simulink model "Hibrido2"  (R2015a)
settings: Solver=ode45  StartTime=0.0  StopTime=1  RelTol=1e-3
values from neighbouring files (symbols this model uses):
  T = 1    [Variaveis.mat]
settings Model: Creator=Afonso  LastModifiedBy=Élio

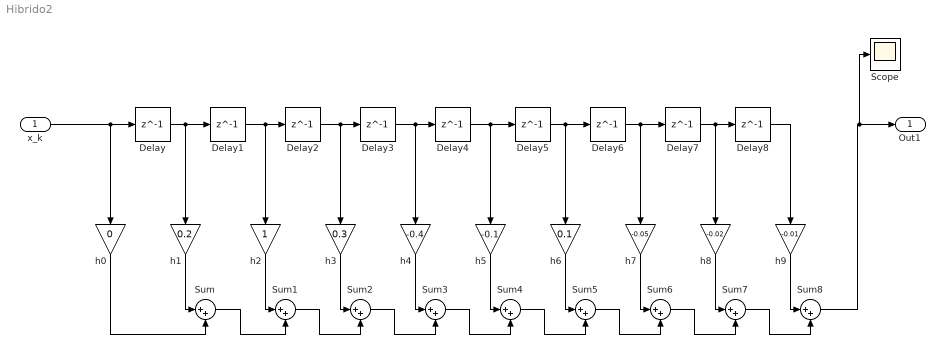
== system Hibrido2 ==
  x_k : Inport
  Delay{,1..8} (9 alike) : Delay  DelayLength=1  SampleTime=T
  Scope : Scope
  Sum{,1..8} (9 alike) : Sum  Inputs=|++
  h0 : Gain  Gain=0
  h1 : Gain  Gain=0.2
  h2 : Gain
  h3 : Gain  Gain=0.3
  h4 : Gain  Gain=-0.4
  h5 : Gain  Gain=-0.1
  h6 : Gain  Gain=0.1
  h7 : Gain  Gain=-0.05
  h8 : Gain  Gain=-0.02
  h9 : Gain  Gain=-0.01
  Out1 : Outport
  wires:
  Sum5/1 -> Sum6/2
  Sum1/1 -> Sum2/2
  Sum6/1 -> Sum7/2
  h9/1 -> Sum8/1
  Sum4/1 -> Sum5/2
  Sum7/1 -> Sum8/2
  Sum3/1 -> Sum4/2
  Sum8/1 -> Scope/1, Out1/1
  Sum2/1 -> Sum3/2
  h7/1 -> Sum6/1
  h8/1 -> Sum7/1
  Delay1/1 -> Delay2/1, h2/1
  Delay/1 -> Delay1/1, h1/1
  Delay2/1 -> Delay3/1, h3/1
  Delay3/1 -> Delay4/1, h4/1
  Delay4/1 -> Delay5/1, h5/1
  Delay6/1 -> Delay7/1, h7/1
  Sum/1 -> Sum1/2
  h2/1 -> Sum1/1
  Delay8/1 -> h9/1
  h1/1 -> Sum/1
  Delay7/1 -> Delay8/1, h8/1
  x_k/1 -> Delay/1, h0/1
  h0/1 -> Sum/2
  h4/1 -> Sum3/1
  h5/1 -> Sum4/1
  Delay5/1 -> Delay6/1, h6/1
  h3/1 -> Sum2/1
  h6/1 -> Sum5/1
